simulink model "as2_dynamics"  (R2024a)
settings: Solver=VariableStepAuto  StartTime=0.0  StopTime=10  RelTol=1e-3
settings Model: Creator=mike_wang  LastModifiedBy=mike_wang

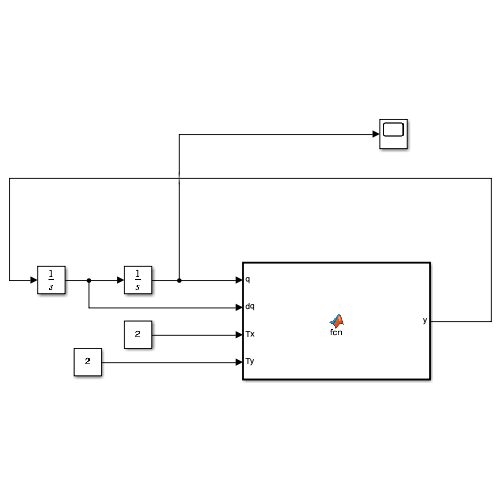
[thumbnail: Simulink's stored preview of the top-level diagram]
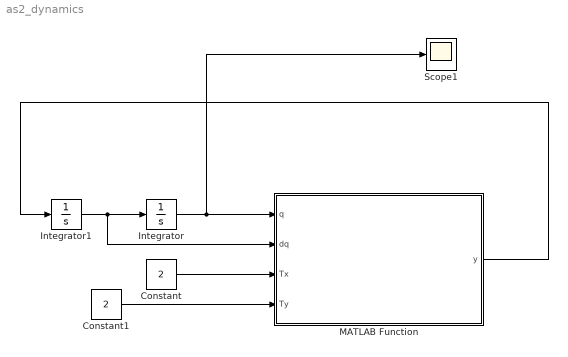
== system as2_dynamics ==
  Constant : Constant  Value=2
  Constant1 : Constant  Value=2
  Integrator : Integrator  InitialCondition=[0;0]
  Integrator1 : Integrator  InitialCondition=[0;0]
  MATLAB Function : MATLAB Function  TreatAsAtomicUnit=on
  Scope1 : Scope
  wires:
  Integrator/1 -> Scope1/1, MATLAB Function/1(q)
  Integrator1/1 -> MATLAB Function/2(dq), Integrator/1
  MATLAB Function/1(y) -> Integrator1/1
  Constant/1 -> MATLAB Function/3(Tx)
  Constant1/1 -> MATLAB Function/4(Ty)

== matlab function as2_dynamics/MATLAB Function ==
  data: q input; y output; dq input; Tx input; Ty input
function y=fcn(q,dq,Tx,Ty)
    m1=2;m2=4;l1=0.6;l2=0.4;
    lc1=l1/2;lc2=l2/2;
    I1=m1*l1^2/3;
    I2=m2*l2^2/3;
    g=9.8;

    p1=m1*lc1^2+m2*l1^2+I1;
    p2=m2*lc2^2+I2;
    p3=m2*l1*lc2;
    p4=m1*lc1+m2*l1;
    p5=m2*lc2;

    D=[[p1+p2+2*p3*cos(q(2)),p2+p3*cos(q(2))];
        [p2+p3*cos(q(2)),p2]];
    C=[[-p3*dq(2)*sin(q(2)),-p3*(dq(1)+dq(2))*sin(q(2))];
        [p3*dq(1)*sin(q(2)),0]];
    G=[p4*g*cos(q(1))+p5*g*cos(q(1)+q(2));p5*g*cos(q(1)+q(2))];

    u=D^(-1)*([Tx;Ty]-C*q-G);

y = u;
